simulink model "Simulateur_V7_eq06"  (R2025b)
settings: Solver=FixedStepAuto  StartTime=0.0  StopTime=5  FixedStep=0.0001  RelTol=1e-3
model workspace (MAT data in the model file):
  B = 0.1128
  Br = 1.2
  D = 0.002
  E = 18600000000
  Filt = 0.09
  GainAmpliPuissance = 1.86
  L = 0.246
  N = 66
  R = 0.016
  T = Simulink.LookupTable
  T.Table = Simulink.lookuptable.Table
  T.Table.Dimensions = [0 0]
  T.Table.DataType = 'auto'
  T.Table.FieldName = 'Table'
  T.Breakpoints = Simulink.lookuptable.Breakpoint
  T.Breakpoints.TunableSizeName = 'N1'
  T.Breakpoints.TunableSizeValue = -1
  T.Breakpoints.Dimensions = [0 0]
  T.Breakpoints.DataType = 'auto'
  T.Breakpoints.FieldName = 'BP1'
  T.AllowMultipleInstancesOfTypeToHaveDifferentTableBreakpointSizes = 0
  T.SupportTunableSize = 0
  T.StructTypeInfo = Simulink.lookuptable.StructTypeInfo
  T.StructTypeInfo.DataScope = 'Auto'
  b = 0.06
  c = 0.43454
  cap = -0.111
  dens = 1850
  freq = 0.00204081632653
  h = 0.00156
  m = 0.1
  m_supp = 0.03
  q = 0.135
  r = 0.0203
  temp_add = 6
libraries: simulink x3, slpidlib x2
settings Model: SimulationMode=accelerator  Creator=jeann
settings RTWCC: GPUComputeCapability=3.5

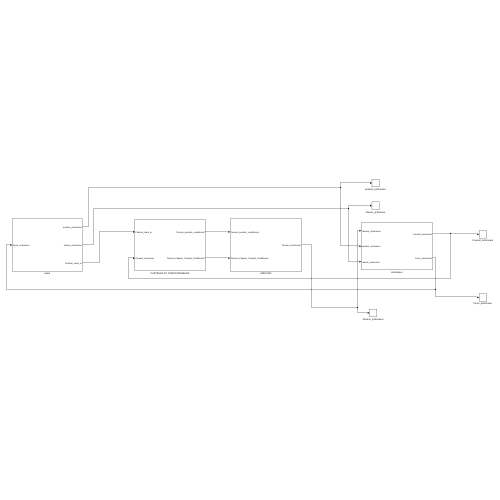
[thumbnail: Simulink's stored preview of the top-level diagram]
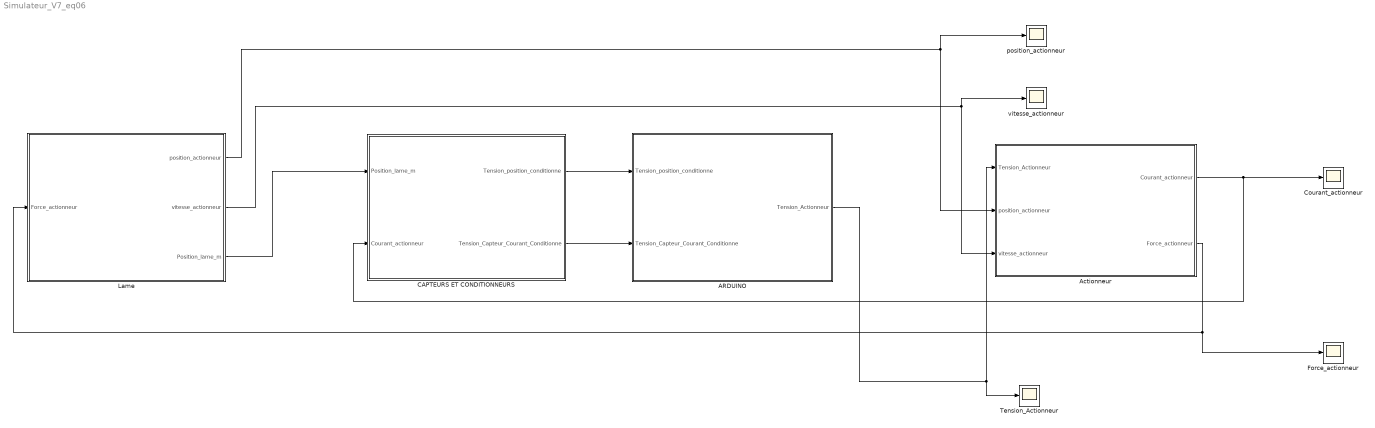
== system Simulateur_V7_eq06 ==
  ARDUINO : Subsystem
  Actionneur : Subsystem
  CAPTEURS ET CONDITIONNEURS : Subsystem
  Courant_actionneur : Scope
      settings: DataLoggingVariableName=ScopeData6
  Force_actionneur : Scope
      settings: DataLoggingVariableName=ScopeData7
  Lame : Subsystem
  Tension_Actionneur : Scope
      settings: DataLoggingVariableName=ScopeData4
  position_actionneur : Scope
  vitesse_actionneur : Scope
      settings: DataLoggingVariableName=ScopeData2
  wires:
  Lame/1(position_actionneur) -> position_actionneur/1, Actionneur/2(position_actionneur)
  Lame/2(vitesse_actionneur) -> Actionneur/3(vitesse_actionneur), vitesse_actionneur/1
  Lame/3(Position_lame_m) -> CAPTEURS ET CONDITIONNEURS/1(Position_lame_m)
  CAPTEURS ET CONDITIONNEURS/1(Tension_position_conditionne) -> ARDUINO/1(Tension_position_conditionne)
  CAPTEURS ET CONDITIONNEURS/2(Tension_Capteur_Courant_Conditionne) -> ARDUINO/2(Tension_Capteur_Courant_Conditionne)
  ARDUINO/1(Tension_Actionneur) -> Tension_Actionneur/1, Actionneur/1(Tension_Actionneur)
  Actionneur/1(Courant_actionneur) -> Courant_actionneur/1, CAPTEURS ET CONDITIONNEURS/2(Courant_actionneur)
  Actionneur/2(Force_actionneur) -> Lame/1(Force_actionneur), Force_actionneur/1

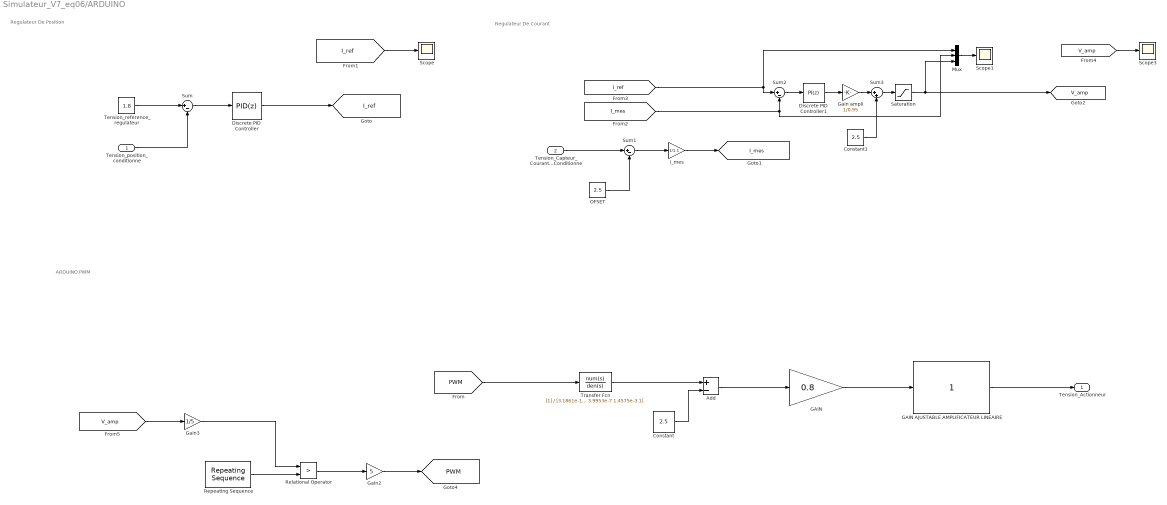
== system Simulateur_V7_eq06/ARDUINO ==
  note: Regulateur De Position
  note: Regulateur De Courant
  note: ARDUINO PWM
  Tension_position_conditionne : Inport
  Tension_Capteur_Courant_Conditionne : Inport  Port=2
  Add : Sum  Inputs=+-
  Constant : Constant  Value=2.5
  Constant1 : Constant  Value=2.5
  Discrete PID Controller : slpidlib/PID Controller  Controller=PID  Form=Parallel  TimeDomain=Discrete-time  UseExternalTs=off  SampleTime=0.002  IntegratorMethod=Forward Euler  FilterMethod=Forward Euler  ControllerParametersSource=internal  P=0.85  I=2.8333  UseKiTs=off  D=0.017  UseExternalDerivativeSource=off  N=100  UseFilter=on  TunerSelectOption=Transfer Function Based (PID Tuner App)  InitialConditionSource=internal  InitialConditionForIntegrator=0  InitialConditionForFilter=0  DifferentiatorICPrevScaledInput=0  ExternalReset=none  TrackingMode=off  Kt=1  LimitOutput=on  SatLimitsSource=internal  UpperSaturationLimit=2.9  LowerSaturationLimit=-2.9  LinearizeAsGain=off  AntiWindupMode=back-calculation  Kb=1  LimitIntegrator=off  UpperIntegratorSaturationLimit=inf  LowerIntegratorSaturationLimit=-inf  POutMin=[]  POutMax=[]  IOutMin=[]  IOutMax=[]  DOutMin=[]  DOutMax=[]  NOutMin=[]  NOutMax=[]  SumOutMin=[]  SumOutMax=[]  SaturationOutMin=[]  SaturationOutMax=[]  PParamMin=[]  PParamMax=[]  IParamMin=[]  IParamMax=[]  DParamMin=[]  DParamMax=[]  NParamMin=[]  NParamMax=[]  KbParamMin=[]  KbParamMax=[]  KtParamMin=[]  KtParamMax=[]  KbOutMin=[]  KbOutMax=[]  KtOutMin=[]  KtOutMax=[]  IntegratorOutMin=[]  IntegratorOutMax=[]  FilterOutMin=[]  FilterOutMax=[]  SumI1OutMin=[]  SumI1OutMax=[]  SumI2OutMin=[]  SumI2OutMax=[]  SumI3OutMin=[]  SumI3OutMax=[]  SumI4OutMin=[]  SumI4OutMax=[]  SumDOutMin=[]  SumDOutMax=[]  DifferentiatorOutMin=[]  DifferentiatorOutMax=[]  FilterDiffOutCoefMin=[]  FilterDiffOutCoefMax=[]  ReciprocalOutMin=[]  ReciprocalOutMax=[]  SumDenOutMin=[]  SumDenOutMax=[]  SumNumOutMin=[]  SumNumOutMax=[]  DivideOutMin=[]  DivideOutMax=[]  UdiffTsProdOutMin=[]  UdiffTsProdOutMax=[]  NTsProdOutMin=[]  NTsProdOutMax=[]  UintegralTsProdOutMin=[]  UintegralTsProdOutMax=[]  UngainTsProdOutMin=[]  UngainTsProdOutMax=[]  ClampingZeroOutDataTypeStr=Inherit: Inherit via back propagation  ClampingZeroOutMin=[]  ClampingZeroOutMax=[]  FilterDenConstantOutDataTypeStr=Inherit: Inherit via back propagation  FilterDenConstantOutMin=[]  FilterDenConstantOutMax=[]  PCopyOutDataTypeStr=Inherit: Inherit via back propagation  PCopyOutMin=[]  PCopyOutMax=[]  NCopyOutDataTypeStr=Inherit: Inherit via back propagation  NCopyOutMin=[]  NCopyOutMax=[]  IntegratorContinuousStateAttributes=''  IntegratorStateMustResolveToSignalObject=off  IntegratorRTWStateStorageClass=Auto  FilterContinuousStateAttributes=''  FilterStateMustResolveToSignalObject=off  FilterRTWStateStorageClass=Auto  ParallelPVariant=InternalParameters  IdealPVariant=Disabled  IVariant=InternalParameters  DVariant=InternalParameters  IntegratorVariant=Discrete  SatVariant=Enabled  AWVariant=BackCalculation  PCopyVariant=Disabled  TRVariant=Disabled  FdbkBlocksVariant=Forward  IdealPFdbkVariant=Disabled  SatFdbkVariant=Disabled  DerivativeFilterVariant=ForwardEulerFilter  NVariant=InternalParameters  NCopyVariant=Disabled  FilterICVariant=InternalICsFilter  IntegratorICVariant=InternalICs  ExternalResetVariant=Disabled  TRSumVariant=Passthrough  SumFdbkVariant=Disabled  SumVariant=Sum_PID  TsampFilterVariant=InternalTs  TsampNgainVariant=Passthrough  TsampIntegralVariant=Disabled_SignalSpec  ExternalSaturationOutDataTypeStr=Inherit: Same as second input  DerivativeSourceVariant=ErrorSignal  PreIntVariant=InternalPreInt
      settings: LibrarySourceBlock=simulink/Discrete/Discrete PID Controller
  Discrete PID Controller1 : slpidlib/PID Controller  Controller=PI  Form=Parallel  TimeDomain=Discrete-time  UseExternalTs=off  SampleTime=0.002  IntegratorMethod=Forward Euler  FilterMethod=Forward Euler  ControllerParametersSource=internal  P=0.18  I=180  UseKiTs=off  D=0  UseExternalDerivativeSource=off  N=100  UseFilter=on  TunerSelectOption=Transfer Function Based (PID Tuner App)  InitialConditionSource=internal  InitialConditionForIntegrator=0  InitialConditionForFilter=0  DifferentiatorICPrevScaledInput=0  ExternalReset=none  TrackingMode=off  Kt=1  LimitOutput=on  SatLimitsSource=internal  UpperSaturationLimit=5  LowerSaturationLimit=0  LinearizeAsGain=off  AntiWindupMode=back-calculation  Kb=1  LimitIntegrator=off  UpperIntegratorSaturationLimit=inf  LowerIntegratorSaturationLimit=-inf  POutMin=[]  POutMax=[]  IOutMin=[]  IOutMax=[]  DOutMin=[]  DOutMax=[]  NOutMin=[]  NOutMax=[]  SumOutMin=[]  SumOutMax=[]  SaturationOutMin=[]  SaturationOutMax=[]  PParamMin=[]  PParamMax=[]  IParamMin=[]  IParamMax=[]  DParamMin=[]  DParamMax=[]  NParamMin=[]  NParamMax=[]  KbParamMin=[]  KbParamMax=[]  KtParamMin=[]  KtParamMax=[]  KbOutMin=[]  KbOutMax=[]  KtOutMin=[]  KtOutMax=[]  IntegratorOutMin=[]  IntegratorOutMax=[]  FilterOutMin=[]  FilterOutMax=[]  SumI1OutMin=[]  SumI1OutMax=[]  SumI2OutMin=[]  SumI2OutMax=[]  SumI3OutMin=[]  SumI3OutMax=[]  SumI4OutMin=[]  SumI4OutMax=[]  SumDOutMin=[]  SumDOutMax=[]  DifferentiatorOutMin=[]  DifferentiatorOutMax=[]  FilterDiffOutCoefMin=[]  FilterDiffOutCoefMax=[]  ReciprocalOutMin=[]  ReciprocalOutMax=[]  SumDenOutMin=[]  SumDenOutMax=[]  SumNumOutMin=[]  SumNumOutMax=[]  DivideOutMin=[]  DivideOutMax=[]  UdiffTsProdOutMin=[]  UdiffTsProdOutMax=[]  NTsProdOutMin=[]  NTsProdOutMax=[]  UintegralTsProdOutMin=[]  UintegralTsProdOutMax=[]  UngainTsProdOutMin=[]  UngainTsProdOutMax=[]  ClampingZeroOutDataTypeStr=Inherit: Inherit via back propagation  ClampingZeroOutMin=[]  ClampingZeroOutMax=[]  FilterDenConstantOutDataTypeStr=Inherit: Inherit via back propagation  FilterDenConstantOutMin=[]  FilterDenConstantOutMax=[]  PCopyOutDataTypeStr=Inherit: Inherit via back propagation  PCopyOutMin=[]  PCopyOutMax=[]  NCopyOutDataTypeStr=Inherit: Inherit via back propagation  NCopyOutMin=[]  NCopyOutMax=[]  IntegratorContinuousStateAttributes=''  IntegratorStateMustResolveToSignalObject=off  IntegratorRTWStateStorageClass=Auto  FilterContinuousStateAttributes=''  FilterStateMustResolveToSignalObject=off  FilterRTWStateStorageClass=Auto  ParallelPVariant=InternalParameters  IdealPVariant=Disabled  IVariant=InternalParameters  DVariant=Disabled  IntegratorVariant=Discrete  SatVariant=Enabled  AWVariant=BackCalculation  PCopyVariant=Disabled  TRVariant=Disabled  FdbkBlocksVariant=Forward  IdealPFdbkVariant=Disabled  SatFdbkVariant=Disabled  DerivativeFilterVariant=Disabled  NVariant=Disabled  NCopyVariant=Disabled_SignalSpec  FilterICVariant=Disabled  IntegratorICVariant=InternalICs  ExternalResetVariant=Disabled  TRSumVariant=Passthrough  SumFdbkVariant=Disabled  SumVariant=Sum_PI  TsampFilterVariant=InternalTs  TsampNgainVariant=Passthrough  TsampIntegralVariant=Disabled_SignalSpec  ExternalSaturationOutDataTypeStr=Inherit: Same as second input  DerivativeSourceVariant=Disabled  PreIntVariant=InternalPreInt
      settings: LibrarySourceBlock=simulink/Discrete/Discrete PID Controller
  GAIN : Gain  Gain=0.8
  GAIN AJUSTABLE AMPLIFICATEUR LINEAIRE : simulink/Math Operations/Slider Gain  gain=1  low=1  high=5
  "Gain ampli " : Gain  Gain=1/0.95
  Gain2 : Gain  Gain=5  ParamDataTypeStr=double
  Gain3 : Gain  Gain=1/5
  Mux : Mux  Inputs=3
  OFSET : Constant  Value=2.5
  Relational Operator : RelationalOperator  Operator=>  OutDataTypeStr=boolean  RndMeth=Simplest  InputSameDT=off
  Repeating Sequence : simulink/Sources/Repeating Sequence  rep_seq_t=[0 0.001 0.002]  rep_seq_y=[0 1 0]
  Saturation : Saturate  UpperLimit=5  LowerLimit=0
  Scope : Scope
      settings: ActiveDisplayYMinimum=-2.2667783988706121  ActiveDisplayYMaximum=-0.54885366678041059  DataLoggingVariableName=ScopeData11
  Scope1 : Scope
      settings: ActiveDisplayYMinimum=-4.3071689204474479  ActiveDisplayYMaximum=3.85630162846556
  Scope3 : Scope
      settings: ActiveDisplayYMinimum=2.2778244916208985  ActiveDisplayYMaximum=2.7526074548655841  DataLoggingVariableName=ScopeData13
  Sum : Sum  Inputs=|+-
  Sum1 : Sum  Inputs=|+-
  Sum2 : Sum  Inputs=|+-
  Sum3 : Sum  Inputs=|++
  Tension_reference_regulateur : Constant  Value=1.8
  Transfer Fcn : TransferFcn  Denominator=[3.1861e-12 3.9953e-7 1.4575e-3 1]
  i_mes : Gain  Gain=1/1.1
  Tension_Actionneur : Outport
  tag scope: I_mes=global, I_ref=global, PWM=global, V_amp=global
  wires:
  Tension_position_conditionne/1 -> Sum/2
  Tension_reference_regulateur/1 -> Sum/1
  [I_ref] -> Scope/1
  Sum/1 -> Discrete PID Controller/1
  Discrete PID Controller/1 -> [I_ref]
  Mux/1 -> Scope1/1
  Sum1/1 -> i_mes/1
  Discrete PID Controller1/1 -> "Gain ampli "/1
  "Gain ampli "/1 -> Sum3/1
  Sum2/1 -> Discrete PID Controller1/1
  i_mes/1 -> [I_mes]
  [I_ref] -> Sum2/1, Mux/1
  Sum3/1 -> Saturation/1
  [V_amp] -> Scope3/1
  OFSET/1 -> Sum1/2
  [I_mes] -> Mux/2, Sum2/2
  Constant1/1 -> Sum3/2
  Saturation/1 -> [V_amp], Mux/3
  Tension_Capteur_Courant_Conditionne/1 -> Sum1/1
  Gain2/1 -> [PWM]
  Gain3/1 -> Relational Operator/1
  [PWM] -> Transfer Fcn/1
  Repeating Sequence/1 -> Relational Operator/2
  Relational Operator/1 -> Gain2/1
  [V_amp] -> Gain3/1
  GAIN AJUSTABLE AMPLIFICATEUR LINEAIRE/1 -> Tension_Actionneur/1
  Transfer Fcn/1 -> Add/1
  GAIN/1 -> GAIN AJUSTABLE AMPLIFICATEUR LINEAIRE/1
  Add/1 -> GAIN/1
  Constant/1 -> Add/2

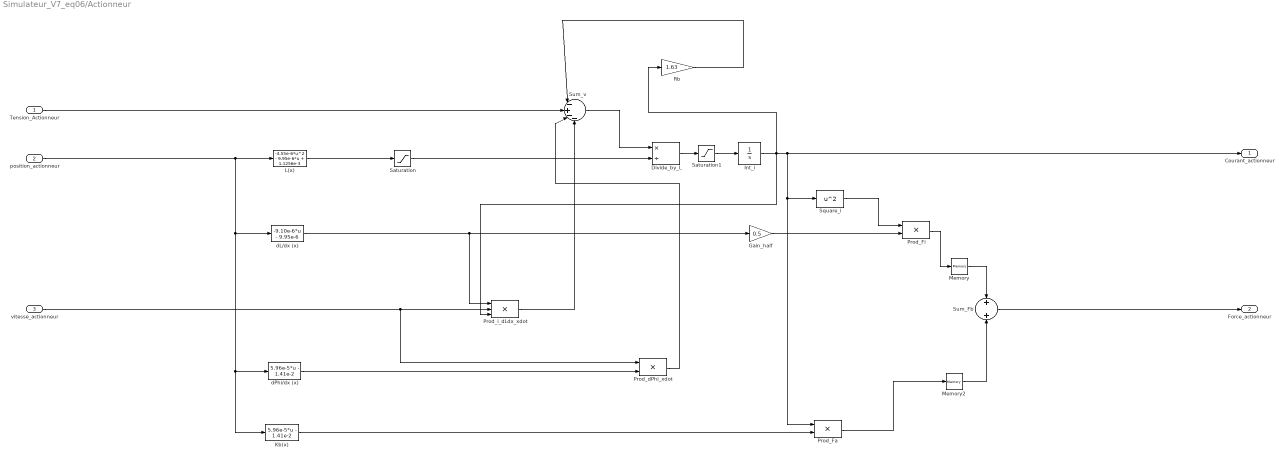
== system Simulateur_V7_eq06/Actionneur ==
  Tension_Actionneur : Inport
  position_actionneur : Inport  Port=2
  vitesse_actionneur : Inport  Port=3
  Divide_by_L : Product  Inputs=*/
  Gain_half : Gain  Gain=0.5
  Int_i : Integrator
  Kb(x) : Fcn  Expr=5.96e-5*u - 1.41e-2
  L(x) : Fcn  Expr=-4.55e-6*u^2 - 9.95e-6*u + 1.1256e-3
  Memory : Memory
  Memory2 : Memory
  Prod_Fa : Product
  Prod_Fi : Product
  Prod_dPhi_xdot : Product
  Prod_i_dLdx_xdot : Product  Inputs=3
  Rb : Gain  Gain=1.63
  Saturation : Saturate  UpperLimit=1  LowerLimit=2e-4
  Saturation1 : Saturate  UpperLimit=1e4  LowerLimit=-1e4
  Square_i : Math  Operator=square
  Sum_Fb : Sum
  Sum_v : Sum  Inputs=|-+--
  dL/dx (x) : Fcn  Expr=-9.10e-6*u - 9.95e-6
  dPhi/dx (x) : Fcn  Expr=5.96e-5*u - 1.41e-2
  Courant_actionneur : Outport
  Force_actionneur : Outport  Port=2
  wires:
  dL/dx (x)/1 -> Gain_half/1, Prod_i_dLdx_xdot/1
  Sum_Fb/1 -> Force_actionneur/1
  Rb/1 -> Sum_v/1
  Prod_i_dLdx_xdot/1 -> Sum_v/4
  L(x)/1 -> Saturation/1
  Square_i/1 -> Prod_Fi/1
  Prod_dPhi_xdot/1 -> Sum_v/3
  Gain_half/1 -> Prod_Fi/2
  dPhi/dx (x)/1 -> Prod_dPhi_xdot/2
  Divide_by_L/1 -> Saturation1/1
  Int_i/1 -> Prod_i_dLdx_xdot/3, Courant_actionneur/1, Square_i/1, Prod_Fa/1, Rb/1
  Sum_v/1 -> Divide_by_L/1
  vitesse_actionneur/1 -> Prod_dPhi_xdot/1, Prod_i_dLdx_xdot/2
  Kb(x)/1 -> Prod_Fa/2
  position_actionneur/1 -> dL/dx (x)/1, Kb(x)/1, dPhi/dx (x)/1, L(x)/1
  Tension_Actionneur/1 -> Sum_v/2
  Prod_Fi/1 -> Memory/1
  Memory/1 -> Sum_Fb/1
  Prod_Fa/1 -> Memory2/1
  Memory2/1 -> Sum_Fb/2
  Saturation/1 -> Divide_by_L/2
  Saturation1/1 -> Int_i/1

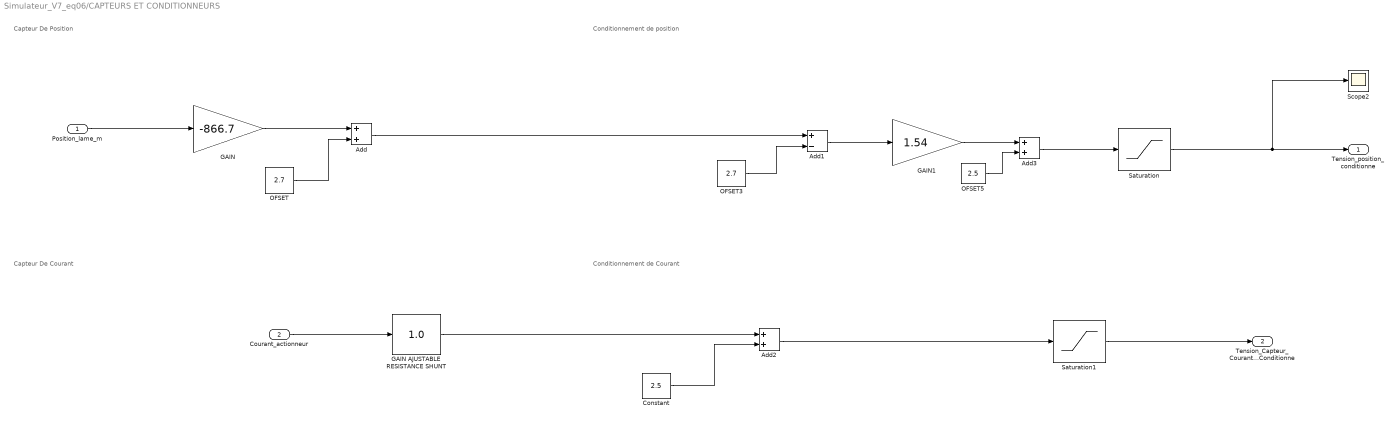
== system Simulateur_V7_eq06/CAPTEURS ET CONDITIONNEURS ==
  note: Capteur De Position
  note: Conditionnement de position
  note: Capteur De Courant
  note: Conditionnement de Courant
  Position_lame_m : Inport
  Courant_actionneur : Inport  Port=2
  Add : Sum
  Add1 : Sum  Inputs=+-
  Add2 : Sum
  Add3 : Sum
  Constant : Constant  Value=2.5
  GAIN : Gain  Gain=-866.7
  GAIN AJUSTABLE RESISTANCE SHUNT : simulink/Math Operations/Slider Gain  gain=1.0  low=1  high=10
  GAIN1 : Gain  Gain=1.54
  OFSET : Constant  Value=2.7
  OFSET3 : Constant  Value=2.7
  OFSET5 : Constant  Value=2.5
  Saturation : Saturate  UpperLimit=5  LowerLimit=0
  Saturation1 : Saturate  UpperLimit=5  LowerLimit=0
  Scope2 : Scope
      settings: ActiveDisplayYMinimum=2.4960699258700285  ActiveDisplayYMaximum=2.5040469319141816  DataLoggingVariableName=ScopeData3
  Tension_position_conditionne : Outport
  Tension_Capteur_Courant_Conditionne : Outport  Port=2
  wires:
  GAIN/1 -> Add/1
  Position_lame_m/1 -> GAIN/1
  Add/1 -> Add1/1
  Add1/1 -> GAIN1/1
  Saturation/1 -> Scope2/1, Tension_position_conditionne/1
  GAIN1/1 -> Add3/1
  OFSET/1 -> Add/2
  OFSET3/1 -> Add1/2
  Courant_actionneur/1 -> GAIN AJUSTABLE RESISTANCE SHUNT/1
  GAIN AJUSTABLE RESISTANCE SHUNT/1 -> Add2/1
  Constant/1 -> Add2/2
  Add2/1 -> Saturation1/1
  Saturation1/1 -> Tension_Capteur_Courant_Conditionne/1
  Add3/1 -> Saturation/1
  OFSET5/1 -> Add3/2

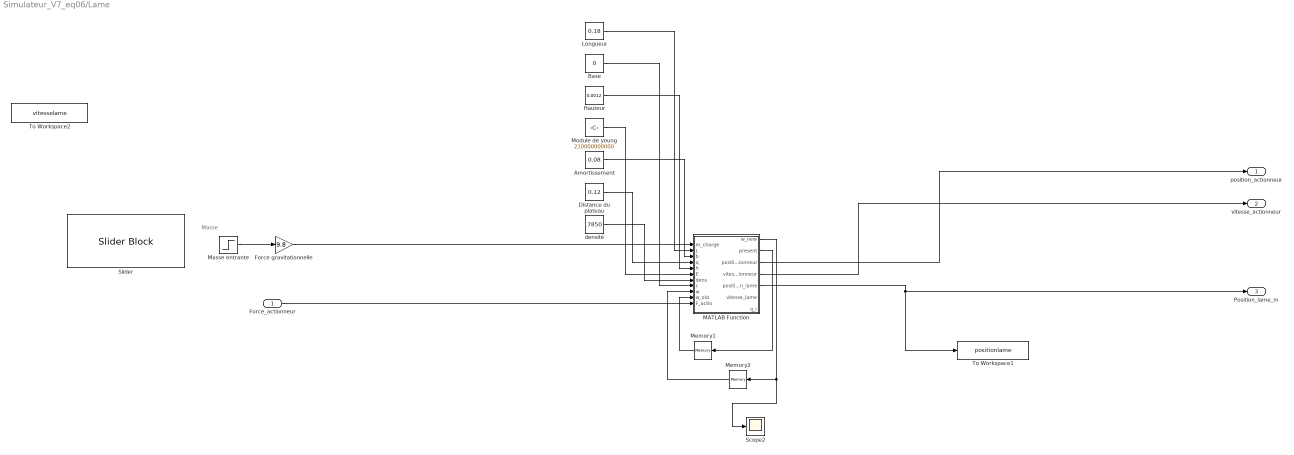
== system Simulateur_V7_eq06/Lame ==
  note: Masse
  Force_actionneur : Inport
  Amortissement : Constant  Value=0.08
  Base : Constant  Value=0
  Distance du plateau : Constant  Value=0.12
  Force gravitationnelle : Gain  Gain=9.8
  Hauteur : Constant  Value=0.0012
  Longueur : Constant  Value=0.18
  MATLAB Function : MATLAB Function  TreatAsAtomicUnit=on
  Masse entrante : Step  After=m  SampleTime=3
  Memory1 : Memory  InitialCondition=zeros(12,1)
  Memory2 : Memory  InitialCondition=zeros(12,1)  StateName=matrix
  Module de young : Constant  Value=210000000000
  Scope2 : Scope
      settings: ActiveDisplayYMinimum=-0.00038987395244894989  ActiveDisplayYMaximum=0.00029932134407525805
  Slider : SliderBlock
  To Workspace1 : ToWorkspace  VariableName=positionlame  SaveFormat=Structure With Time  SampleTime=-1
  To Workspace2 : ToWorkspace  VariableName=vitesselame  SaveFormat=Structure With Time  SampleTime=-1
  densité : Constant  Value=7850
  position_actionneur : Outport
  vitesse_actionneur : Outport  Port=2
  Position_lame_m : Outport  Port=3
  wires:
  Force_actionneur/1 -> MATLAB Function/11(F_actio)
  MATLAB Function/1(w_new) -> Memory2/1, Scope2/1
  Memory2/1 -> MATLAB Function/9(w)
  MATLAB Function/2(present) -> Memory1/1
  Memory1/1 -> MATLAB Function/10(w_old)
  Hauteur/1 -> MATLAB Function/5(h)
  Module de young/1 -> MATLAB Function/6(E)
  Amortissement/1 -> MATLAB Function/3(b)
  Distance du plateau/1 -> MATLAB Function/4(q)
  densité/1 -> MATLAB Function/7(dens)
  Masse entrante/1 -> Force gravitationnelle/1
  Force gravitationnelle/1 -> MATLAB Function/1(m_charge)
  MATLAB Function/5(position_lame) -> To Workspace1/1, Position_lame_m/1
  MATLAB Function/4(vitesse_actionneur) -> vitesse_actionneur/1
  MATLAB Function/3(position_actionneur) -> position_actionneur/1
  Longueur/1 -> MATLAB Function/2(L)
  Base/1 -> MATLAB Function/8(c)

== matlab function Simulateur_V7_eq06/Lame/MATLAB Function ==
  data: m_charge input; L input; b input; q input; h input; E input; dens input; c input; w_new output; w input; w_old input; present output; position_actionneur output; vitesse_actionneur output; position_lame output; vitesse_lame output; F_actio input; q_i output
function [w_new, present, position_actionneur, vitesse_actionneur, position_lame, vitesse_lame, q_i] = fcn(m_charge, L, b, q, h, E, dens, c, w, w_old, F_actio)

% =========================
% Paramètres de la poutre
% =========================
J = b*h^3/12;          % Moment quadratique de la section [m^4]
mu = dens*b*h;         % Masse linéique [kg/m]

% =========================
% Paramètres physiques
% =========================
m_lame   = mu*L;       % Masse totale approximative de la lame [kg]
m_aimant = 9.3e-3;     % Masse de l'aimant [kg]
g = -9.8;              % Gravité [m/s^2]
dt = 1e-5;             % Pas de temps [s]

% =========================
% Discrétisation spatiale
% =========================
nx = 10;               % Nombre de noeuds internes utiles
dx = L/(nx-1);         % Pas spatial [m]

% Position discrète de la masse / force appliquée
q_i = 2 + round(q/dx);

% Ajout de 2 noeuds fantômes pour les conditions limites
nx = nx + 2;

% Sécurité pour éviter de sortir des bornes utiles
q_i = max(3, min(q_i, nx-2));

% =========================
% Mise en forme des états
% =========================
w     = w(:);
w_old = w_old(:);

if length(w) ~= nx
    w = zeros(nx,1);
end

if length(w_old) ~= nx
    w_old = zeros(nx,1);
end

% =========================
% Vecteur des forces
% =========================
F = zeros(nx,1);
F(end) = g*m_aimant;                 % Poids de l'aimant au bout
F(q_i) = g*m_charge + F_actio;       % Poids de la charge + force actionneur

% =========================
% Coefficients de calcul
% =========================
coeff1   = -E*J*dt^2/(mu*dx^4); % Coefficient de rigidité (flexion de la poutre) : traduit l'effet du terme EI*d^4w/dx^4 sur la déformation
coeff_amt = c*dt/mu;            % Coefficient d’amortissement : modélise les pertes d’énergie (proportionnel à la vitesse (w - w_old))
coeff_F  = dt^2/(mu*dx);        % Coefficient de force : transforme la force appliquée F(i) en déplacement de la lame

% =========================
% Initialisation
% =========================
w_new = zeros(nx,1);

% =========================
% Mise à jour de la déformation
% =========================
i = 3:nx-2;

w_new(i) = ...
    coeff1 * ( w(i+2) - 4*w(i+1) + 6*w(i) - 4*w(i-1) + w(i-2) ) ...
    + 2*w(i) - w_old(i) ...
    - coeff_amt * (w(i) - w_old(i)) ...
    + coeff_F * F(i);

% =========================
% Conditions limites
% =========================
w_new(1:2) = 0;    % Encastrement : déplacement et pente nuls

% Extrémité libre : dérivées 2e et 3e nulles
w_new(end-1) = 2*w_new(end-2) - w_new(end-3);
w_new(end)   = 2*w_new(end-1) - w_new(end-2);

% =========================
% Sorties
% =========================
present = w;                                      % Etat actuel pour mémoire

% Sorties pour l'actionneur (au noeud q_i)
position_actionneur = w_new(q_i);                 
vitesse_actionneur  = (w_new(q_i) - w(q_i))/dt;  

% Sorties pour le capteur de position (au bout de la lame)
position_lame = w_new(end);                       
vitesse_lame  = (w_new(end) - w(end))/dt;         

end
